simulink model "rosberrypi_subscribe_camera"  (R2018b)
settings: Solver=VariableStepAuto  StartTime=0.0  StopTime=inf  RelTol=1e-3  EnableMultiTasking=on
model workspace (MAT data in the model file):
  SL_ROS_VariableLengthArrays_MaxSizes.CommonInfo.ArrayTruncateAction = 'EmitWarning'
  SL_ROS_VariableLengthArrays_MaxSizes.MsgTypeMap = containers.Map
  SL_ROS_VariableLengthArrays_MaxSizes.MsgTypeMap.serialization.keys = {'sensor_msgs/Image'}
  SL_ROS_VariableLengthArrays_MaxSizes.MsgTypeMap.serialization.values{1}(1).PropertyName = 'Encoding'
  SL_ROS_VariableLengthArrays_MaxSizes.MsgTypeMap.serialization.values{1}(1).DataType = 'uint8'
  SL_ROS_VariableLengthArrays_MaxSizes.MsgTypeMap.serialization.values{1}(1).MaxLength = 5
  SL_ROS_VariableLengthArrays_MaxSizes.MsgTypeMap.serialization.values{1}(2).PropertyName = 'Data'
  SL_ROS_VariableLengthArrays_MaxSizes.MsgTypeMap.serialization.values{1}(2).DataType = 'uint8'
  SL_ROS_VariableLengthArrays_MaxSizes.MsgTypeMap.serialization.values{1}(2).MaxLength = 19200
  SL_ROS_VariableLengthArrays_MaxSizes.MsgTypeMap.serialization.uniformity = 0
  SL_ROS_VariableLengthArrays_MaxSizes.MsgTypeMap.serialization.keyType = 'char'
  SL_ROS_VariableLengthArrays_MaxSizes.MsgTypeMap.serialization.valueType = 'any'
libraries: visiongeotforms x1, embdlinuxlib x1, robotlib x1
settings Model: Creator=The MathWorks, Inc.  LastModifiedBy=The MathWorks, Inc.
settings DataIOCC: SaveFormat=Array
settings OptimizationCC: LifeSpan=inf
settings DebuggingCC: SolverPrmCheckMsg=warning  AllowSymbolicDim=off  SFUnexpectedBacktrackingDiag=warning  SFNoUnconditionalDefaultTransitionDiag=warning
settings ModelReferenceCC: PropagateSignalLabelsOutOfModel=off
settings SFSimCC: SimUseLocalCustomCode=off
settings RTWCC: RTWUseLocalCustomCode=off
settings CodeAppCC: StateflowObjectComments=on
settings GRTTargetCC: TargetLangStandard=C89/C90 (ANSI)  GeneratePreprocessorConditionals=Disable all
settings ConfigComp: CovMetricSettings=dw  CovHtmlReporting=on  CovSaveCumulativeToWorkspaceVar=on  CovSaveSingleToWorkspaceVar=on  CovExternalEMLEnable=off  CovSFcnEnable=off

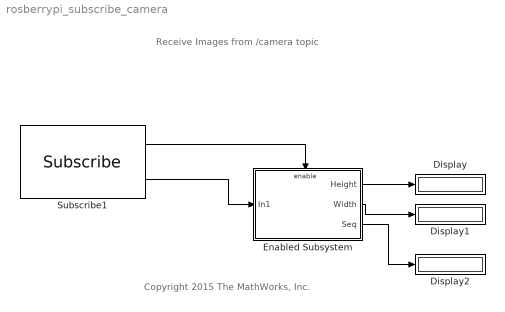
== system rosberrypi_subscribe_camera ==
  note: Receive Images  from
      |  /camera topic
  note: Copyright 2015 The MathWorks, Inc.
  Display : Display
  Display1 : Display
  Display2 : Display
  Enabled Subsystem : Subsystem
  Subscribe1 : robotlib/Subscribe  topicSource=Specify your own  topic=/camera  messageType=sensor_msgs/Image  sampleTime=1/5  messageQueueLength=51
      settings: SourceProductBaseCode=RO
  wires:
  Subscribe1/1 -> Enabled Subsystem/Enable
  Subscribe1/2 -> Enabled Subsystem/1(In1)
  Enabled Subsystem/1(Height) -> Display/1
  Enabled Subsystem/2(Width) -> Display1/1
  Enabled Subsystem/3(Seq) -> Display2/1

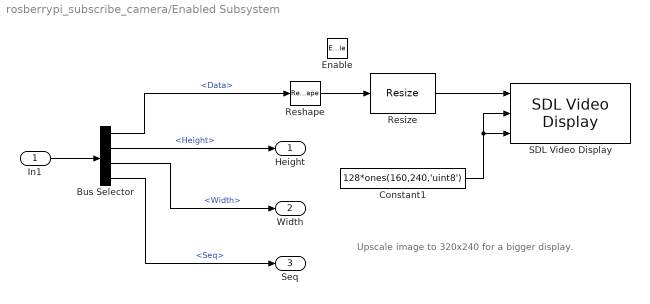
== system rosberrypi_subscribe_camera/Enabled Subsystem ==
  note: Upscale image to 320x240 for a bigger display.
  In1 : Inport
  Enable : EnablePort
  Bus Selector : BusSelector  DialogController=Simulink.DDGSource_BusSelector  OutputSignals=Data,Height,Width,Header.Seq
  Constant1 : Constant  Value=128*ones(160,240,'uint8')
  Reshape : Reshape  OutputDimensionality=Customize  OutputDimensions=[160,120]
  Resize : visiongeotforms/Resize  specify=Output size as a percentage of input size  rfactor=[200 200]  outCols=25  outRows=25  outRowsCols=[25 35]  interp_method=Lanczos2  antialias=on  useROI=off  roiFlag=off  prodOutputMode=Binary point scaling  prodOutputWordLength=32  prodOutputFracLength=10  roundingMode=Nearest  overflowMode=on
      settings: SourceProductName=Computer Vision System Toolbox  SourceProductBaseCode=VP
  SDL Video Display : embdlinuxlib/SDL Video Display  pixelFormat=YCbCr 4:2:2  pixelOrder=Planar  rowMajor=on  blockPlatform=Raspberry Pi
      settings: SourceProductName=Simulink Support Package for Raspberry Pi Hardware  SourceProductBaseCode=RASPPI
  Height : Outport
  Width : Outport  Port=2
  Seq : Outport  Port=3
  wires:
  In1/1 -> Bus Selector/1
  Bus Selector/3 -> Width/1  "<Width>"
  Bus Selector/2 -> Height/1  "<Height>"
  Bus Selector/1 -> Reshape/1  "<Data>"
  Reshape/1 -> Resize/1
  Constant1/1 -> SDL Video Display/3, SDL Video Display/2
  Bus Selector/4 -> Seq/1  "<Seq>"
  Resize/1 -> SDL Video Display/1
